simulink subsystem "ENVIRONMENT"  (R2025b)
settings: Solver=VariableStepAuto  StartTime=0.0  StopTime=10.0  RelTol=1e-3
undefined symbols (not defined in the file): WMM2025
libraries: simulink_extras x2, aerolibgravity2 x2, aerolibtransform2 x1, aerolibatmos2 x1
settings Model: Creator=antoniohernandez-rodiciomateos  LastModifiedBy=antoniohernandez-rodiciomateos

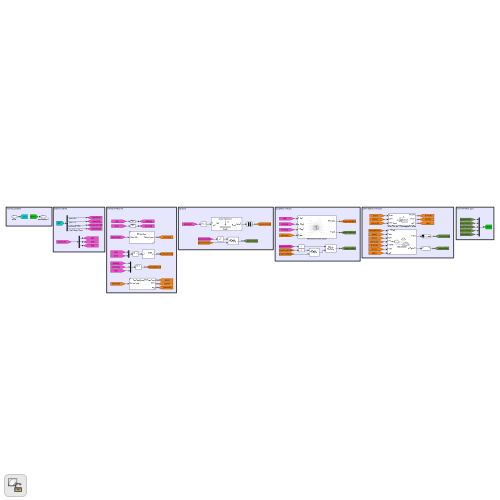
[thumbnail: Simulink's stored preview of the top-level diagram]
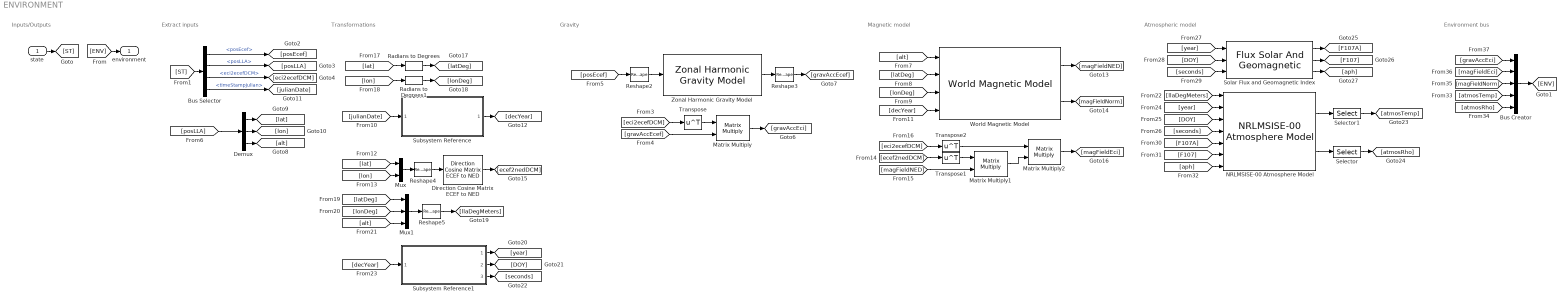
== system ENVIRONMENT ==
  note: Gravity
  note: Extract inputs
  note: Inputs/Outputs
  note: Transformations
  note: Magnetic model
  note: Atmospheric model
  note: Environment bus
  state : Inport  OutDataTypeStr=Bus: state_bus
  Bus Creator : BusCreator  Inputs=5  OutDataTypeStr=Bus: environment_bus  NonVirtualBus=on
      settings: InheritFromInputs=off
  Bus Selector : BusSelector  OutputSignals=posEcef,posLLA,eci2ecefDCM,timeStampJulian
  Demux : Demux  Outputs=3
  Direction Cosine Matrix ECEF to NED : aerolibtransform2/Direction Cosine Matrix ECEF to NED
  Matrix Multiply : Product  Multiplication=Matrix(*)
  Matrix Multiply1 : Product  Multiplication=Matrix(*)
  Matrix Multiply2 : Product  Multiplication=Matrix(*)
  Mux : Mux  Inputs=2
  Mux1 : Mux  Inputs=3
  NRLMSISE-00 Atmosphere Model : aerolibatmos2/NRLMSISE-00 Atmosphere Model  units=Metric (MKS)  lst_input=off  flux_ap_input=on  flags_input=Internal  flags=ones(1,23)  oxygen_in=on  action=Warning
  Radians to Degrees : simulink_extras/Transformations/Radians to Degrees
  Radians to Degrees1 : simulink_extras/Transformations/Radians to Degrees
  Reshape2 : Reshape
  Reshape3 : Reshape  OutputDimensionality=Column vector (2-D)
  Reshape4 : Reshape
  Reshape5 : Reshape
  Selector : Selector  InputPortWidth=9  IndexOptions=Index vector (dialog)  Indices=[6]  OutputSizes=1
  Selector1 : Selector  InputPortWidth=2  IndexOptions=Index vector (dialog)  Indices=[2]  OutputSizes=1
  Solar Flux and Geomagnetic Index : FluxSolarAndGeomagnetic
  Subsystem Reference : Subsystem  ReferencedSubsystem=jd2decYear
  Subsystem Reference1 : Subsystem  ReferencedSubsystem=decYear2yearDOYsec
  Transpose : Math  Operator=transpose
  Transpose1 : Math  Operator=transpose
  Transpose2 : Math  Operator=transpose
  World Magnetic Model : aerolibgravity2/World Magnetic Model  model=WMM2025 (2025-2030)  customFile='WMM2025.COF'  units=Metric (MKS)  time_in=on  month=January  day=1  year=2025  action=Error  h_out=off  dec_out=off  inc_out=off  ti_out=on
  Zonal Harmonic Gravity Model : aerolibgravity2/Zonal Harmonic Gravity Model  units=Metric (MKS)  degree=4  action=Warning  ptype=Earth  R=6378136.3  GM=398600441500000  jvalue=[1.0826269e-03 -2.5323000e-06 -1.6204000e-06]
  environment : Outport  OutDataTypeStr=Bus: environment_bus
  wires:
  state/1 -> [ST]
  [ENV] -> environment/1
  [ST] -> Bus Selector/1
  Bus Selector/1 -> [posEcef]  "<posEcef>"
  Bus Selector/2 -> [posLLA]  "<posLLA>"
  Bus Selector/3 -> [eci2ecefDCM]  "<eci2ecefDCM>"
  [eci2ecefDCM] -> Transpose/1
  Transpose/1 -> Matrix Multiply/1
  [gravAccEcef] -> Matrix Multiply/2
  Matrix Multiply/1 -> [gravAccEci]
  Zonal Harmonic Gravity Model/1 -> Reshape3/1
  Reshape3/1 -> [gravAccEcef]
  Reshape2/1 -> Zonal Harmonic Gravity Model/1
  [posEcef] -> Reshape2/1
  [posLLA] -> Demux/1
  [alt] -> World Magnetic Model/1
  [latDeg] -> World Magnetic Model/2
  [lonDeg] -> World Magnetic Model/3
  Bus Selector/4 -> [julianDate]  "<timeStampJulian>"
  [julianDate] -> Subsystem Reference/1
  Subsystem Reference/1 -> [decYear]
  [decYear] -> World Magnetic Model/4
  World Magnetic Model/1 -> [magFieldNED]
  World Magnetic Model/2 -> [magFieldNorm]
  [lat] -> Mux/1
  [lon] -> Mux/2
  Mux/1 -> Reshape4/1
  Reshape4/1 -> Direction Cosine Matrix ECEF to NED/1
  Direction Cosine Matrix ECEF to NED/1 -> [ecef2nedDCM]
  [ecef2nedDCM] -> Transpose1/1
  Transpose1/1 -> Matrix Multiply1/1
  [magFieldNED] -> Matrix Multiply1/2
  [eci2ecefDCM] -> Transpose2/1
  Matrix Multiply1/1 -> Matrix Multiply2/2
  Transpose2/1 -> Matrix Multiply2/1
  Matrix Multiply2/1 -> [magFieldEci]
  [lat] -> Radians to Degrees/1
  [lon] -> Radians to Degrees1/1
  Radians to Degrees/1 -> [latDeg]
  Radians to Degrees1/1 -> [lonDeg]
  [latDeg] -> Mux1/1
  [lonDeg] -> Mux1/2
  [alt] -> Mux1/3
  Mux1/1 -> Reshape5/1
  Reshape5/1 -> [llaDegMeters]
  [llaDegMeters] -> NRLMSISE-00 Atmosphere Model/1
  [decYear] -> Subsystem Reference1/1
  Subsystem Reference1/1 -> [year]
  Subsystem Reference1/2 -> [DOY]
  Subsystem Reference1/3 -> [seconds]
  [year] -> NRLMSISE-00 Atmosphere Model/2
  [DOY] -> NRLMSISE-00 Atmosphere Model/3
  [seconds] -> NRLMSISE-00 Atmosphere Model/4
  [year] -> Solar Flux and Geomagnetic Index/1
  [DOY] -> Solar Flux and Geomagnetic Index/2
  [seconds] -> Solar Flux and Geomagnetic Index/3
  Solar Flux and Geomagnetic Index/1 -> [F107A]
  Solar Flux and Geomagnetic Index/2 -> [F107]
  Solar Flux and Geomagnetic Index/3 -> [aph]
  [F107A] -> NRLMSISE-00 Atmosphere Model/5
  [F107] -> NRLMSISE-00 Atmosphere Model/6
  [aph] -> NRLMSISE-00 Atmosphere Model/7
  NRLMSISE-00 Atmosphere Model/2 -> Selector/1
  Selector/1 -> [atmosRho]
  NRLMSISE-00 Atmosphere Model/1 -> Selector1/1
  Selector1/1 -> [atmosTemp]
  [magFieldEci] -> Bus Creator/2
  [magFieldNorm] -> Bus Creator/3
  [atmosTemp] -> Bus Creator/4
  [gravAccEci] -> Bus Creator/1
  [atmosRho] -> Bus Creator/5
  Bus Creator/1 -> [ENV]
  Demux/1 -> [lat]
  Demux/2 -> [lon]
  Demux/3 -> [alt]
